simulink model "PLR_final"  (R2023a)
settings: Solver=ode23tb  StartTime=0.0  StopTime=0.05  MaxStep=1e-7  MinStep=1e-8  RelTol=1e-6
libraries: spsVoltageMeasurementLib x27, spsCurrentMeasurementLib x19, spsSeriesRLCBranchLib x15, spsDiodeLib x12, spsGroundLib x9, spsDCVoltageSourceLib x6, spsMosfetLib x6, simulink x4, spsMeanLib x2, sps_lib x1
settings Model: Creator=nikos  LastModifiedBy=nikos

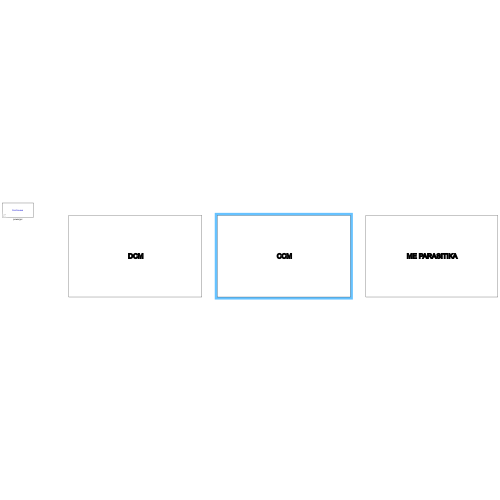
[thumbnail: Simulink's stored preview of the top-level diagram]
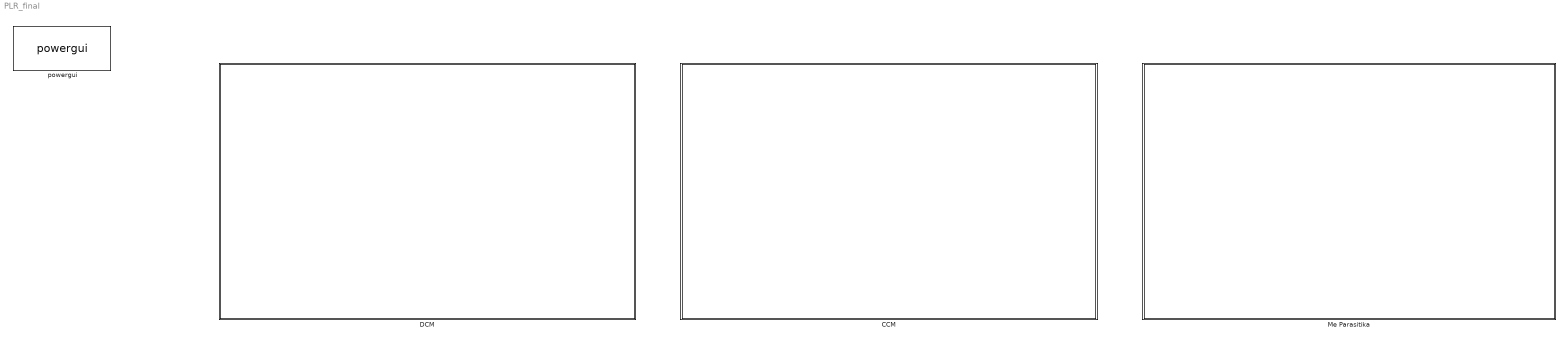
== system PLR_final ==
  CCM : Subsystem
      settings: OpenFcn=open_system(gcb, 'force')
      mask Display: disp('{\bf\fontsize{30}CCM}', 'texmode','on');
  DCM : Subsystem
      settings: OpenFcn=open_system(gcb, 'force')
      mask Display: disp('{\bf\fontsize{30}DCM}', 'texmode','on');
  Me Parasitika : Subsystem
      settings: OpenFcn=open_system(gcb, 'force')
      mask Display: disp('{\bf\fontsize{30}ME PARASITIKA}', 'texmode','on');
  powergui : sps_lib/powergui  Priority=1  SimulationMode=Continuous  SampleTime=50e-6  frequency=60  Iterations=50  frequencyindice=0  Pbase=100e6  ErrMax=1e-4  UnitsV=kV  UnitsW=MW  buscounter=0  FunctionMessages=off  echomessages=off  EnableUseOfTLC=off  CurrentSourceSwitches=off  DisableSnubberDevices=on  DisableRonSwitches=off  DisableVfSwitches=off  DisplayEquations=off  AutomaticDiscreteSolvers=off  SolverType=Tustin/Backward Euler (TBE)  Interpol=off  ExternalGateDelay=off  methode=off  Ts=100  x0status=blocks  SPID=on  SwTol=0  HookPort=off  NonlinearTolerance=1e-4  nMaxIteration=100  ContinueOnMaxIteration=off  RestoreLinks=warning  ResistiveCurrentMeasurement=off  Frange=[0:2:500]  Ylog=off  Xlog=on  ShowGrid=off  save=off  variable=ZData  structure=0  ZoomFFT=off  StartTime=0.0  cycles=1  DisplayStyle=1  fundamental=60  FreqAxis=off  MaxFrequency=1000  frequencyindicesteady=1  RmsSteady=1  display=off

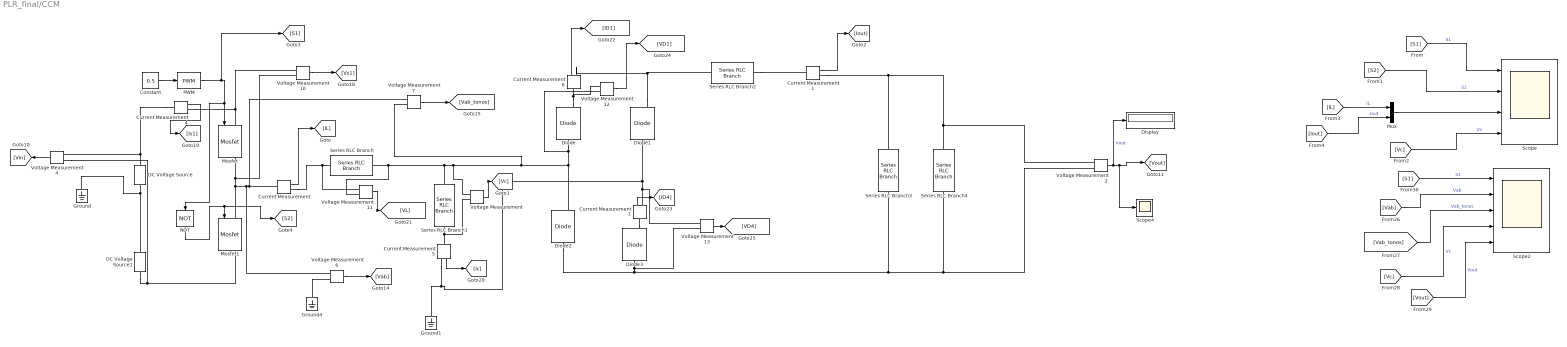
== system PLR_final/CCM ==
  Constant : Constant  Value=0.5
  Current Measurement{,1,4..7} (6 alike) : spsCurrentMeasurementLib/Current Measurement  PhasorSimulation=off  OutputType=Complex  PSBequivalent=0
  DC Voltage Source : spsDCVoltageSourceLib/DC Voltage Source  Amplitude=100  Measurements=None
  DC Voltage Source1 : spsDCVoltageSourceLib/DC Voltage Source  Amplitude=100  Measurements=None
  Diode{,1..3} (4 alike) : spsDiodeLib/Diode  Ron=0.001  Lon=0  Vf=0.8  IC=0  UseSnubber=0  Rs=500  Cs=250e-9  Measurements=on
  Display : Display
  Ground : spsGroundLib/Ground  LConnTagsString=a
  Ground1 : spsGroundLib/Ground  LConnTagsString=a
  Ground4 : spsGroundLib/Ground  LConnTagsString=a
  Mosfet : spsMosfetLib/Mosfet  Ron=0.1  Lon=0  Rd=0.01  Vfd=0  IC=0  Rs=1e5  Cs=inf  Measurements=on
  Mosfet1 : spsMosfetLib/Mosfet  Ron=0.1  Lon=0  Rd=0.01  Vfd=0  IC=0  Rs=1e5  Cs=inf  Measurements=on
  Mux : Mux  Inputs=2
  NOT : Logic  Operator=NOT  IconShape=distinctive  AllPortsSameDT=off  OutDataTypeStr=boolean
  PWM : simulink/Discontinuities/PWM  DisableCoverage=on  Period=1/10000  InitialDelay=0  DisallowZeroDutyCycle=off  RunAtFixedTimeIntervals=off  SampleTime=0.1
  Scope : Scope  NumInputPorts=4
  Scope2 : Scope  NumInputPorts=5
  Scope4 : Scope
  Series RLC Branch : spsSeriesRLCBranchLib/Series RLC Branch  LConnTagsString=__new0  RConnTagsString=__new0  BranchType=L  Resistance=1  Inductance=61.5e-6  SetiL0=off  InitialCurrent=0  Capacitance=1e-6  Setx0=off  InitialVoltage=0  Measurements=None
  Series RLC Branch1 : spsSeriesRLCBranchLib/Series RLC Branch  LConnTagsString=__new0  RConnTagsString=__new0  BranchType=C  Resistance=1  Inductance=1e-3  SetiL0=off  InitialCurrent=0  Capacitance=(100/61.5)*1e-6  Setx0=off  InitialVoltage=0  Measurements=None
  Series RLC Branch2 : spsSeriesRLCBranchLib/Series RLC Branch  LConnTagsString=__new0  RConnTagsString=__new0  BranchType=L  Resistance=1  Inductance=36e-3  SetiL0=off  InitialCurrent=0  Capacitance=1e-6  Setx0=off  InitialVoltage=0  Measurements=None
  Series RLC Branch3 : spsSeriesRLCBranchLib/Series RLC Branch  LConnTagsString=__new0  RConnTagsString=__new0  BranchType=C  Resistance=1  Inductance=1e-3  SetiL0=off  InitialCurrent=0  Capacitance=10e-6  Setx0=off  InitialVoltage=0  Measurements=None
  Series RLC Branch4 : spsSeriesRLCBranchLib/Series RLC Branch  LConnTagsString=__new0  RConnTagsString=__new0  BranchType=R  Resistance=10  Inductance=1e-3  SetiL0=off  InitialCurrent=0  Capacitance=1e-6  Setx0=off  InitialVoltage=0  Measurements=None
  Voltage Measurement{,2,4,6..7,10..13} (9 alike) : spsVoltageMeasurementLib/Voltage Measurement  PhasorSimulation=off  OutputType=Complex  PSBequivalent=0
  wires:
  Voltage Measurement11/1 -> [VL]
  Voltage Measurement6/1 -> [Vab]
  Voltage Measurement2/1 -> Display/1, Scope4/1, [Vout]  "Vout"
  [Vab_tonos] -> Scope2/3  "Vab_tonos"
  [S1] -> Scope2/1  "S1"
  [Vc] -> Scope/4  "Vc"
  PWM/1 -> [S1], NOT/1, Mosfet/1
  Voltage Measurement7/1 -> [Vab_tonos]
  [S1] -> Scope/1  "S1"
  [IL] -> Mux/1  "IL"
  Current Measurement1/1 -> [Iout]
  [Vout] -> Scope2/5  "Vout"
  [Vab] -> Scope2/2  "Vab"
  Current Measurement4/1 -> [Is1]
  Voltage Measurement12/1 -> [VD1]
  [Vc] -> Scope2/4  "Vc"
  Voltage Measurement4/1 -> [Vin]
  Current Measurement7/1 -> [ID4]
  Current Measurement/1 -> [IL]
  Voltage Measurement13/1 -> [VD4]
  Current Measurement5/1 -> [Ic]
  Current Measurement6/1 -> [ID1]
  Voltage Measurement10/1 -> [Vs1]
  [S2] -> Scope/2  "S2"
  Constant/1 -> PWM/1
  Voltage Measurement/1 -> [Vc]
  Mux/1 -> Scope/3
  [Iout] -> Mux/2  "Iout"
  NOT/1 -> [S2], Mosfet1/1
  connections:
  Ground/LConn1 -- DC Voltage Source/LConn1 -- DC Voltage Source1/RConn1
  Diode/RConn1 -- Voltage Measurement12/LConn1 -- Current Measurement6/LConn1
  Series RLC Branch2/RConn1 -- Current Measurement1/LConn1
  Current Measurement4/LConn1 -- Voltage Measurement4/LConn1 -- DC Voltage Source/RConn1
  Current Measurement1/RConn1 -- Series RLC Branch3/LConn1 -- Series RLC Branch4/LConn1 -- Voltage Measurement2/LConn1
  Current Measurement5/LConn1 -- Series RLC Branch1/RConn1 -- Voltage Measurement/LConn2
  Voltage Measurement12/LConn2 -- Diode/LConn1 -- Diode2/RConn1 -- Series RLC Branch1/LConn1 -- Voltage Measurement11/LConn2 -- Series RLC Branch/RConn1 -- Voltage Measurement/LConn1 -- Voltage Measurement7/LConn2
  Current Measurement4/RConn1 -- Mosfet/LConn1 -- Voltage Measurement10/LConn1
  Voltage Measurement4/LConn2 -- Mosfet1/RConn1 -- DC Voltage Source1/LConn1
  Diode1/RConn1 -- Current Measurement6/RConn1 -- Series RLC Branch2/LConn1
  Ground1/LConn1 -- Current Measurement5/RConn1 -- Diode1/LConn1 -- Voltage Measurement13/LConn1 -- Current Measurement7/RConn1
  Current Measurement7/LConn1 -- Diode3/RConn1
  Voltage Measurement6/LConn2 -- Ground4/LConn1
  Voltage Measurement11/LConn1 -- Series RLC Branch/LConn1 -- Current Measurement/RConn1
  Voltage Measurement7/LConn1 -- Current Measurement/LConn1 -- Voltage Measurement6/LConn1 -- Voltage Measurement10/LConn2 -- Mosfet/RConn1 -- Mosfet1/LConn1
  Voltage Measurement2/LConn2 -- Series RLC Branch4/RConn1 -- Series RLC Branch3/RConn1 -- Diode2/LConn1 -- Voltage Measurement13/LConn2 -- Diode3/LConn1

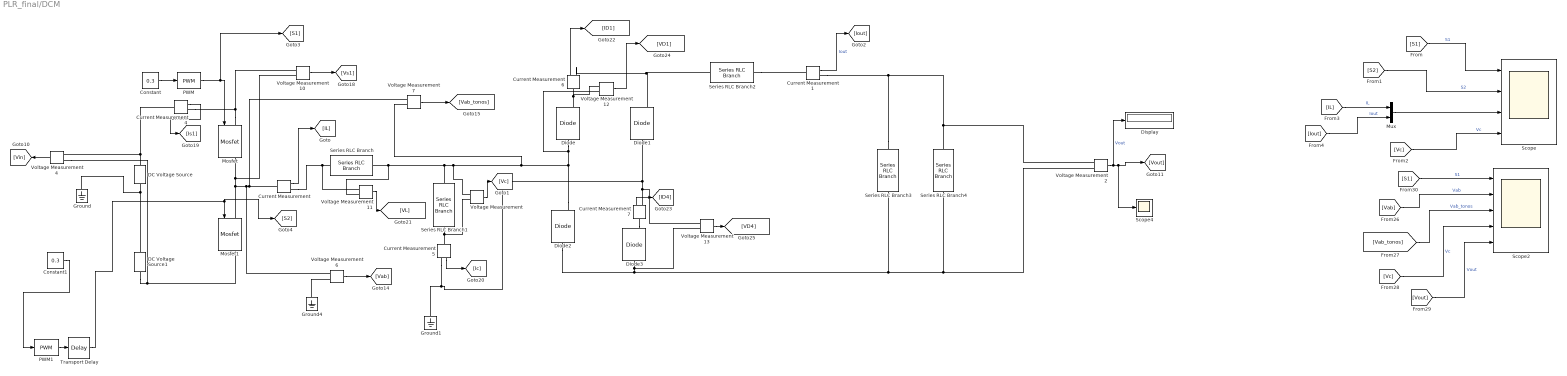
== system PLR_final/DCM ==
  Constant : Constant  Value=0.3
  Constant1 : Constant  Value=0.3
  Current Measurement{,1,4..7} (6 alike) : spsCurrentMeasurementLib/Current Measurement  PhasorSimulation=off  OutputType=Complex  PSBequivalent=0
  DC Voltage Source : spsDCVoltageSourceLib/DC Voltage Source  Amplitude=100  Measurements=None
  DC Voltage Source1 : spsDCVoltageSourceLib/DC Voltage Source  Amplitude=100  Measurements=None
  Diode{,1..3} (4 alike) : spsDiodeLib/Diode  Ron=0.001  Lon=0  Vf=0.8  IC=0  UseSnubber=0  Rs=500  Cs=250e-9  Measurements=on
  Display : Display
  Ground : spsGroundLib/Ground  LConnTagsString=a
  Ground1 : spsGroundLib/Ground  LConnTagsString=a
  Ground4 : spsGroundLib/Ground  LConnTagsString=a
  Mosfet : spsMosfetLib/Mosfet  Ron=0.1  Lon=0  Rd=0.01  Vfd=0  IC=0  Rs=1e5  Cs=inf  Measurements=on
  Mosfet1 : spsMosfetLib/Mosfet  Ron=0.1  Lon=0  Rd=0.01  Vfd=0  IC=0  Rs=1e5  Cs=inf  Measurements=on
  Mux : Mux  Inputs=2
  PWM : simulink/Discontinuities/PWM  DisableCoverage=on  Period=1/5000  InitialDelay=0  DisallowZeroDutyCycle=off  RunAtFixedTimeIntervals=off  SampleTime=0.1
  PWM1 : simulink/Discontinuities/PWM  DisableCoverage=on  Period=1/5000  InitialDelay=0  DisallowZeroDutyCycle=off  RunAtFixedTimeIntervals=off  SampleTime=0.1
  Scope : Scope  NumInputPorts=4
  Scope2 : Scope  NumInputPorts=5
  Scope4 : Scope
  Series RLC Branch : spsSeriesRLCBranchLib/Series RLC Branch  LConnTagsString=__new0  RConnTagsString=__new0  BranchType=L  Resistance=1  Inductance=61.5e-6  SetiL0=off  InitialCurrent=0  Capacitance=1e-6  Setx0=off  InitialVoltage=0  Measurements=None
  Series RLC Branch1 : spsSeriesRLCBranchLib/Series RLC Branch  LConnTagsString=__new0  RConnTagsString=__new0  BranchType=C  Resistance=1  Inductance=1e-3  SetiL0=off  InitialCurrent=0  Capacitance=(100/61.5)*1e-6  Setx0=off  InitialVoltage=0  Measurements=None
  Series RLC Branch2 : spsSeriesRLCBranchLib/Series RLC Branch  LConnTagsString=__new0  RConnTagsString=__new0  BranchType=L  Resistance=1  Inductance=36e-3  SetiL0=off  InitialCurrent=0  Capacitance=1e-6  Setx0=off  InitialVoltage=0  Measurements=None
  Series RLC Branch3 : spsSeriesRLCBranchLib/Series RLC Branch  LConnTagsString=__new0  RConnTagsString=__new0  BranchType=C  Resistance=1  Inductance=1e-3  SetiL0=off  InitialCurrent=0  Capacitance=10e-6  Setx0=off  InitialVoltage=0  Measurements=None
  Series RLC Branch4 : spsSeriesRLCBranchLib/Series RLC Branch  LConnTagsString=__new0  RConnTagsString=__new0  BranchType=R  Resistance=10  Inductance=1e-3  SetiL0=off  InitialCurrent=0  Capacitance=1e-6  Setx0=off  InitialVoltage=0  Measurements=None
  Transport Delay : TransportDelay  DelayTime=0.5/5000
  Voltage Measurement{,2,4,6..7,10..13} (9 alike) : spsVoltageMeasurementLib/Voltage Measurement  PhasorSimulation=off  OutputType=Complex  PSBequivalent=0
  wires:
  Voltage Measurement11/1 -> [VL]
  Voltage Measurement6/1 -> [Vab]
  Voltage Measurement2/1 -> Display/1, Scope4/1, [Vout]  "Vout"
  [Vab_tonos] -> Scope2/3  "Vab_tonos"
  [S1] -> Scope2/1  "S1"
  PWM1/1 -> Transport Delay/1
  [Vc] -> Scope/4  "Vc"
  PWM/1 -> [S1], Mosfet/1
  Voltage Measurement7/1 -> [Vab_tonos]
  [S1] -> Scope/1  "S1"
  [IL] -> Mux/1  "IL"
  Current Measurement1/1 -> [Iout]  "Iout"
  [Vout] -> Scope2/5  "Vout"
  [Vab] -> Scope2/2  "Vab"
  Transport Delay/1 -> [S2], Mosfet1/1
  Constant1/1 -> PWM1/1
  Current Measurement4/1 -> [Is1]
  Voltage Measurement12/1 -> [VD1]
  [Vc] -> Scope2/4  "Vc"
  Voltage Measurement4/1 -> [Vin]
  Current Measurement7/1 -> [ID4]
  Current Measurement/1 -> [IL]
  Voltage Measurement13/1 -> [VD4]
  Current Measurement5/1 -> [Ic]
  Current Measurement6/1 -> [ID1]
  Voltage Measurement10/1 -> [Vs1]
  [S2] -> Scope/2  "S2"
  Constant/1 -> PWM/1
  Voltage Measurement/1 -> [Vc]
  Mux/1 -> Scope/3
  [Iout] -> Mux/2  "Iout"
  connections:
  Ground/LConn1 -- DC Voltage Source1/RConn1 -- DC Voltage Source/LConn1
  Voltage Measurement12/LConn1 -- Current Measurement6/LConn1 -- Diode/RConn1
  Series RLC Branch2/RConn1 -- Current Measurement1/LConn1
  Voltage Measurement4/LConn1 -- DC Voltage Source/RConn1 -- Current Measurement4/LConn1
  Series RLC Branch3/LConn1 -- Series RLC Branch4/LConn1 -- Voltage Measurement2/LConn1 -- Current Measurement1/RConn1
  Series RLC Branch1/RConn1 -- Voltage Measurement/LConn2 -- Current Measurement5/LConn1
  Diode2/RConn1 -- Series RLC Branch1/LConn1 -- Voltage Measurement11/LConn2 -- Series RLC Branch/RConn1 -- Voltage Measurement/LConn1 -- Voltage Measurement7/LConn2 -- Voltage Measurement12/LConn2 -- Diode/LConn1
  Mosfet/LConn1 -- Voltage Measurement10/LConn1 -- Current Measurement4/RConn1
  Mosfet1/RConn1 -- DC Voltage Source1/LConn1 -- Voltage Measurement4/LConn2
  Current Measurement6/RConn1 -- Series RLC Branch2/LConn1 -- Diode1/RConn1
  Current Measurement7/RConn1 -- Ground1/LConn1 -- Current Measurement5/RConn1 -- Diode1/LConn1 -- Voltage Measurement13/LConn1
  Current Measurement7/LConn1 -- Diode3/RConn1
  Voltage Measurement6/LConn2 -- Ground4/LConn1
  Series RLC Branch/LConn1 -- Current Measurement/RConn1 -- Voltage Measurement11/LConn1
  Mosfet/RConn1 -- Voltage Measurement10/LConn2 -- Mosfet1/LConn1 -- Voltage Measurement7/LConn1 -- Current Measurement/LConn1 -- Voltage Measurement6/LConn1
  Series RLC Branch3/RConn1 -- Diode2/LConn1 -- Voltage Measurement13/LConn2 -- Diode3/LConn1 -- Voltage Measurement2/LConn2 -- Series RLC Branch4/RConn1

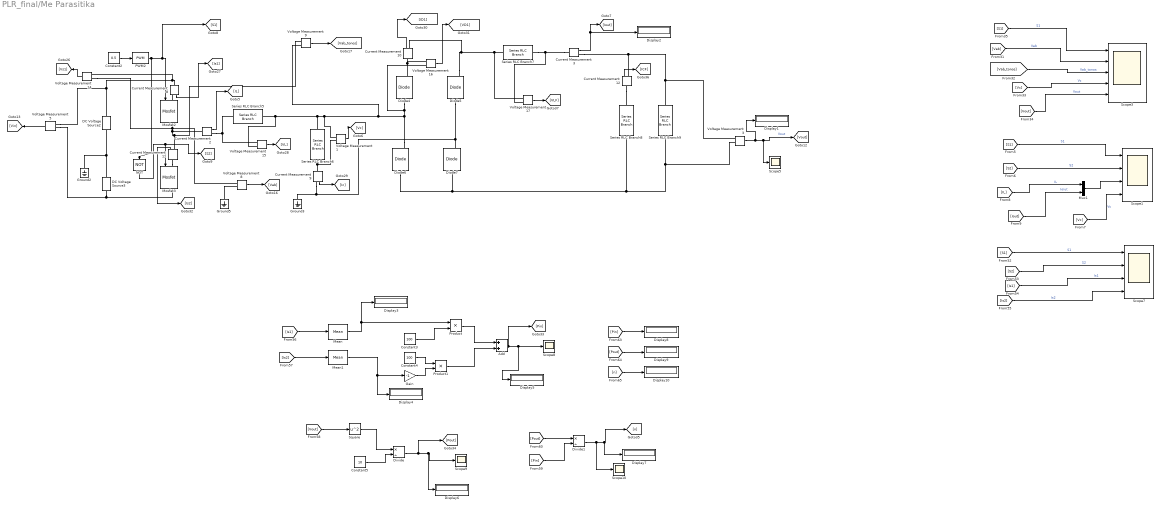
== system PLR_final/Me Parasitika ==
  Add : Sum
  Constant2 : Constant  Value=0.5
  Constant3 : Constant  Value=100
  Constant4 : Constant  Value=100
  Constant5 : Constant  Value=10
  Current Measurement{2..3,8..12} (7 alike) : spsCurrentMeasurementLib/Current Measurement  PhasorSimulation=off  OutputType=Complex  PSBequivalent=0
  DC Voltage Source2 : spsDCVoltageSourceLib/DC Voltage Source  Amplitude=100  Measurements=None
  DC Voltage Source3 : spsDCVoltageSourceLib/DC Voltage Source  Amplitude=100  Measurements=None
  Diode{4..7} (4 alike) : spsDiodeLib/Diode  Ron=0.1e-3  Lon=0  Vf=0.52  IC=0  UseSnubber=0  Rs=500  Cs=250e-9  Measurements=on
  Display{1..10} (10 alike) : Display
  Divide : Product  Inputs=*/
  Divide1 : Product  Inputs=*/
  Gain : Gain  Gain=-1
  Ground2 : spsGroundLib/Ground  LConnTagsString=a
  Ground3 : spsGroundLib/Ground  LConnTagsString=a
  Ground5 : spsGroundLib/Ground  LConnTagsString=a
  Mean : spsMeanLib/Mean  Freq=26420  Vinit=0  Ts=0
  Mean1 : spsMeanLib/Mean  Freq=26420  Vinit=0  Ts=0
  Mosfet2 : spsMosfetLib/Mosfet  Ron=15e-3  Lon=0  Rd=0  Vfd=0  IC=0  Rs=1e5  Cs=inf  Measurements=on
  Mosfet3 : spsMosfetLib/Mosfet  Ron=15e-3  Lon=0  Rd=0  Vfd=0  IC=0  Rs=1e5  Cs=inf  Measurements=on
  Mux1 : Mux  Inputs=2
  NOT : Logic  Operator=NOT  IconShape=distinctive  AllPortsSameDT=off  OutDataTypeStr=boolean
  PWM2 : simulink/Discontinuities/PWM  DisableCoverage=on  Period=1/26420  InitialDelay=0  DisallowZeroDutyCycle=off  RunAtFixedTimeIntervals=off  SampleTime=0.1
  Product : Product
  Product1 : Product
  Scope1 : Scope  NumInputPorts=4
  Scope{5,8..10} (4 alike) : Scope
  Scope3 : Scope  NumInputPorts=5
  Scope7 : Scope  NumInputPorts=4
  Series RLC Branch5 : spsSeriesRLCBranchLib/Series RLC Branch  LConnTagsString=__new0  RConnTagsString=__new0  BranchType=RL  Resistance=48e-3  Inductance=180e-6  SetiL0=off  InitialCurrent=0  Capacitance=1e-6  Setx0=off  InitialVoltage=0  Measurements=None
  Series RLC Branch6 : spsSeriesRLCBranchLib/Series RLC Branch  LConnTagsString=__new0  RConnTagsString=__new0  BranchType=RC  Resistance=0.04e-3  Inductance=1e-3  SetiL0=off  InitialCurrent=0  Capacitance=5.7e-7  Setx0=off  InitialVoltage=0  Measurements=None
  Series RLC Branch7 : spsSeriesRLCBranchLib/Series RLC Branch  LConnTagsString=__new0  RConnTagsString=__new0  BranchType=RL  Resistance=40e-3  Inductance=1e-3  SetiL0=off  InitialCurrent=0  Capacitance=1e-6  Setx0=off  InitialVoltage=0  Measurements=None
  Series RLC Branch8 : spsSeriesRLCBranchLib/Series RLC Branch  LConnTagsString=__new0  RConnTagsString=__new0  BranchType=RC  Resistance=3e-3  Inductance=1e-3  SetiL0=off  InitialCurrent=0  Capacitance=100e-6  Setx0=off  InitialVoltage=0  Measurements=None
  Series RLC Branch9 : spsSeriesRLCBranchLib/Series RLC Branch  LConnTagsString=__new0  RConnTagsString=__new0  BranchType=R  Resistance=10  Inductance=1e-3  SetiL0=off  InitialCurrent=0  Capacitance=1e-6  Setx0=off  InitialVoltage=0  Measurements=None
  Square : Math  Operator=square
  Voltage Measurement{1,3,5,8..9,14..17} (9 alike) : spsVoltageMeasurementLib/Voltage Measurement  PhasorSimulation=off  OutputType=Complex  PSBequivalent=0
  wires:
  Voltage Measurement17/1 -> [VLF]
  [S1] -> Scope3/1  "S1"
  [IL] -> Mux1/1  "IL"
  Current Measurement12/1 -> [ICF]
  Voltage Measurement5/1 -> [Vin]
  Divide1/1 -> Scope10/1, Display7/1, [n]
  [S1] -> Scope1/1  "S1"
  [Pin] -> Display8/1
  Product1/1 -> Add/2
  Add/1 -> [Pin], Display5/1, Scope8/1
  [S1] -> Scope7/1  "S1"
  Current Measurement2/1 -> [IL]
  Gain/1 -> Product1/2
  Constant5/1 -> Divide/2
  Voltage Measurement15/1 -> [VL]
  Constant3/1 -> Product/2
  Voltage Measurement1/1 -> [Vc]
  [Vout] -> Scope3/5  "Vout"
  NOT/1 -> [S2], Mosfet3/1
  Mean/1 -> Display3/1, Product/1
  Mux1/1 -> Scope1/3
  [Is2] -> Mean1/1
  Voltage Measurement9/1 -> [Vab_tonos]
  [n] -> Display10/1
  Voltage Measurement16/1 -> [VD1]
  [Pin] -> Divide1/2
  [S2] -> Scope7/2  "S2"
  Voltage Measurement3/1 -> Display1/1, Scope5/1, [Vout]  "Vout"
  Divide/1 -> [Pout], Display6/1, Scope9/1
  Mean1/1 -> Gain/1, Display4/1
  [Pout] -> Display9/1
  [Vab] -> Scope3/2  "Vab"
  [Is2] -> Scope7/4  "Is2"
  Current Measurement9/1 -> [Ic]
  Product/1 -> Add/1
  [Pout] -> Divide1/1
  Square/1 -> Divide/1
  [Vc] -> Scope3/4  "Vc"
  Voltage Measurement8/1 -> [Vab]
  PWM2/1 -> [S1], Mosfet2/1, NOT/1
  Voltage Measurement14/1 -> [Vs1]
  [Iout] -> Mux1/2  "Ioiut"
  [S2] -> Scope1/2  "S2"
  Current Measurement3/1 -> Display2/1, [Iout]
  [Is1] -> Scope7/3  "Is1"
  [Vout] -> Square/1
  Current Measurement11/1 -> [Is2]
  [Vab_tonos] -> Scope3/3  "Vab_tonos"
  Current Measurement10/1 -> [ID1]
  [Is1] -> Mean/1
  Constant2/1 -> PWM2/1
  Constant4/1 -> Product1/1
  Current Measurement8/1 -> [Is1]
  [Vc] -> Scope1/4  "Vc"
  connections:
  Ground3/LConn1 -- Diode5/LConn1 -- Diode7/RConn1 -- Current Measurement9/RConn1
  Mosfet2/RConn1 -- Voltage Measurement9/LConn1 -- Current Measurement11/RConn1 -- Current Measurement2/LConn1 -- Voltage Measurement14/LConn2 -- Voltage Measurement8/LConn1
  Series RLC Branch6/RConn1 -- Voltage Measurement1/LConn2 -- Current Measurement9/LConn1
  Current Measurement12/LConn1 -- Series RLC Branch8/LConn1
  DC Voltage Source2/LConn1 -- DC Voltage Source3/RConn1 -- Ground2/LConn1
  Voltage Measurement8/LConn2 -- Ground5/LConn1
  Current Measurement8/RConn1 -- Mosfet2/LConn1
  Current Measurement11/LConn1 -- Mosfet3/LConn1
  Voltage Measurement14/LConn1 -- DC Voltage Source2/RConn1 -- Voltage Measurement5/LConn1 -- Current Measurement8/LConn1
  Diode5/RConn1 -- Current Measurement10/RConn1 -- Series RLC Branch7/LConn1 -- Voltage Measurement17/LConn1
  Diode6/RConn1 -- Voltage Measurement16/LConn2 -- Diode4/LConn1 -- Voltage Measurement9/LConn2 -- Voltage Measurement15/LConn2 -- Series RLC Branch5/RConn1 -- Series RLC Branch6/LConn1 -- Voltage Measurement1/LConn1
  Mosfet3/RConn1 -- DC Voltage Source3/LConn1 -- Voltage Measurement5/LConn2
  Current Measurement3/RConn1 -- Voltage Measurement3/LConn1 -- Series RLC Branch9/LConn1 -- Current Measurement12/RConn1
  Voltage Measurement16/LConn1 -- Current Measurement10/LConn1 -- Diode4/RConn1
  Voltage Measurement15/LConn1 -- Current Measurement2/RConn1 -- Series RLC Branch5/LConn1
  Voltage Measurement3/LConn2 -- Series RLC Branch9/RConn1 -- Series RLC Branch8/RConn1 -- Diode6/LConn1 -- Diode7/LConn1
  Current Measurement3/LConn1 -- Series RLC Branch7/RConn1 -- Voltage Measurement17/LConn2
